simulink model "zadacha_12"  (Simulink 7.1)
settings: Solver=ode45  StartTime=0  StopTime=150  RelTol=1e-3
settings Model: Creator=Slavi  LastModifiedBy=Slavi

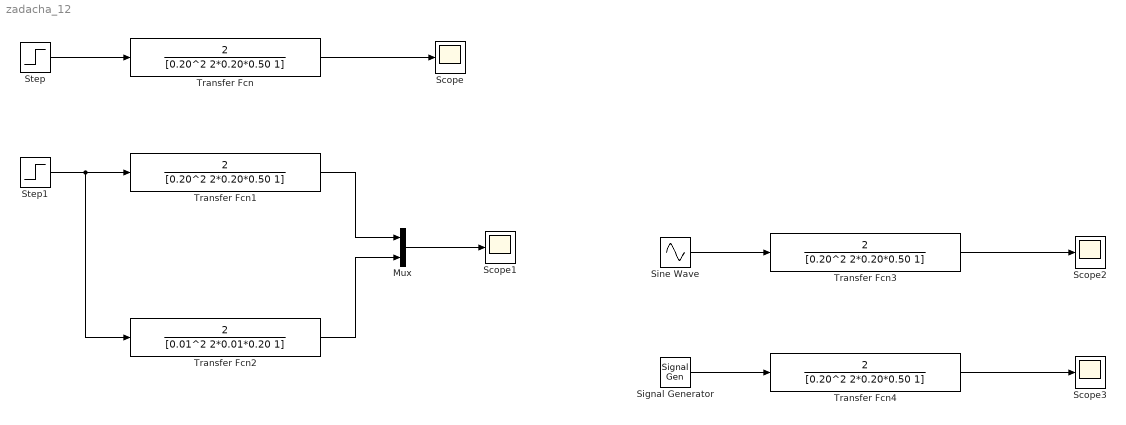
== system zadacha_12 ==
  Mux : Mux  Inputs=2
  Scope{,1..3} (4 alike) : Scope
      Scope2 settings: SaveName=ScopeData2
      Scope3 settings: SaveName=ScopeData3
  Signal Generator : SignalGenerator  WaveForm=square  Frequency=5
  Sine Wave : Sin
  Step : Step
  Step1 : Step
  Transfer Fcn{,1,3..4} (4 alike) : TransferFcn  Numerator=[2]  Denominator=[0.20^2 2*0.20*0.50 1]
  Transfer Fcn2 : TransferFcn  Numerator=[2]  Denominator=[0.01^2 2*0.01*0.20 1]
  wires:
  Transfer Fcn/1 -> Scope/1
  Step/1 -> Transfer Fcn/1
  Step1/1 -> Transfer Fcn1/1, Transfer Fcn2/1
  Transfer Fcn1/1 -> Mux/1
  Transfer Fcn2/1 -> Mux/2
  Mux/1 -> Scope1/1
  Transfer Fcn3/1 -> Scope2/1
  Sine Wave/1 -> Transfer Fcn3/1
  Transfer Fcn4/1 -> Scope3/1
  Signal Generator/1 -> Transfer Fcn4/1
